simulink model "UpdatePulseTime"  (R2020a)
settings: Solver=FixedStepAuto  StartTime=0.0  StopTime=10.0  FixedStep=1e-3  RelTol=1e-3  EnableMultiTasking=on
settings Model: ExtModeTrigDuration=5  Creator=WinnieTrandinh  LastModifiedBy=WinnieTrandinh
settings OptimizationCC: EnhancedBackFolding=on  PassReuseOutputArgsAs=Individual arguments  ZeroExternalMemoryAtStartup=off  ZeroInternalMemoryAtStartup=off  MaxStackSize=64  OptimizeBlockOrder=speed  DifferentSizesBufferReuse=on  OptimizationCustomize=off  EfficientTunableParamExpr=on
settings DebuggingCC: ParameterTunabilityLossMsg=error
settings HardwareCC: ProdBitPerPointer=32  ProdBitPerSizeT=32  ProdBitPerPtrDiffT=32  ProdLargestAtomicInteger=Long  ProdLargestAtomicFloat=Double  ProdWordSize=32  ProdHWDeviceType=ARM Compatible->ARM Cortex
settings SFSimCC: MATLABDynamicMemAlloc=off
settings RTWCC: SystemTargetFile=ert.tlc  HardwareBoard=NXP FRDM-K64F  TemplateMakefile=ert_default_tmf  Toolchain=GNU Tools for ARM Embedded Processors
settings CodeAppCC: ForceParamTrailComments=on  IgnoreCustomStorageClasses=off  OperatorAnnotations=on  SimulinkDataObjDesc=on  SFDataObjDesc=on  InsertBlockDesc=on

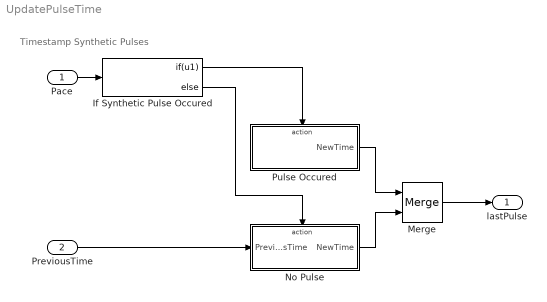
== system UpdatePulseTime ==
  note: Timestamp Synthetic Pulses
  Pace : Inport  OutDataTypeStr=boolean
  PreviousTime : Inport  Port=2
  If Synthetic Pulse Occured : If  IfExpression=u1
  Merge : Merge
  No Pulse : Subsystem  TreatAsAtomicUnit=on
  Pulse Occured : Subsystem  TreatAsAtomicUnit=on
  lastPulse : Outport
  wires:
  If Synthetic Pulse Occured/1 -> Pulse Occured/Action
  Pulse Occured/1(NewTime) -> Merge/1
  No Pulse/1(NewTime) -> Merge/2
  If Synthetic Pulse Occured/2 -> No Pulse/Action
  Pace/1 -> If Synthetic Pulse Occured/1
  Merge/1 -> lastPulse/1
  PreviousTime/1 -> No Pulse/1(PreviousTime)

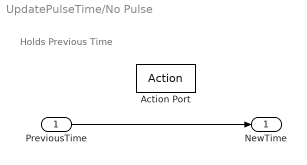
== system UpdatePulseTime/No Pulse ==
  note: Holds Previous Time
  PreviousTime : Inport
  Action Port : ActionPort  ActionPortLabel=else
  NewTime : Outport
  wires:
  PreviousTime/1 -> NewTime/1

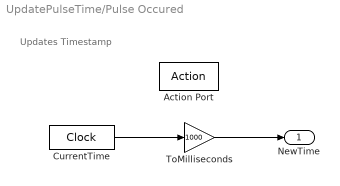
== system UpdatePulseTime/Pulse Occured ==
  note: Updates Timestamp
  Action Port : ActionPort  ActionPortLabel=if(u1)
  CurrentTime : DigitalClock  SampleTime=0.001
  ToMilliseconds : Gain  Gain=1000
  NewTime : Outport
  wires:
  CurrentTime/1 -> ToMilliseconds/1
  ToMilliseconds/1 -> NewTime/1
